simulink model "count_5_constant_2016"  (R2016b)
settings: Solver=VariableStepAuto  StartTime=0.0  StopTime=10.0  RelTol=1e-3
settings Model: Creator=AKSHAY JP PAWAR  LastModifiedBy=AKSHAY JP PAWAR
settings DataIOCC: ReturnWorkspaceOutputs=on
settings SFSimCC: SimUseLocalCustomCode=on
settings RTWCC: RTWUseLocalCustomCode=on

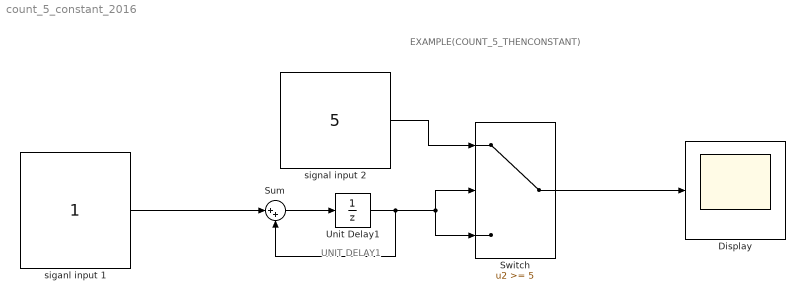
== system count_5_constant_2016 ==
  note: EXAMPLE(COUNT_5_THENCONSTANT)
  note: UNIT DELAY1
  Display : Scope
  Sum : Sum  Inputs=|++
  Switch : Switch  Threshold=5
  Unit Delay1 : UnitDelay  SampleTime=-1  HasFrameUpgradeWarning=on
  siganl input 1 : Constant
  signal input 2 : Constant  Value=5
  wires:
  Sum/1 -> Unit Delay1/1
  signal input 2/1 -> Switch/1
  siganl input 1/1 -> Sum/1
  Switch/1 -> Display/1
  Unit Delay1/1 -> Sum/2, Switch/3, Switch/2
